simulink model "SWC_FDC_type"  (R2021b)
settings: Solver=FixedStepDiscrete  StartTime=0.0  StopTime=10.0  FixedStep=0.005  RelTol=1e-3
values from neighbouring files (symbols this model uses):
  FALSE = boolean( 0 )    [vcu_local_hdr.m]    (also in vcu_local_hdrTA2.m)
  TRUE = boolean( 1 )    [vcu_local_hdr.m]    (also in vcu_local_hdrTA2.m)
libraries: app x1
settings Model: DataDictionary=APPTypes.sldd  Creator=FVT22063  LastModifiedBy=zack
settings DataIOCC: SaveFormat=StructureWithTime
settings OptimizationCC: DefaultParameterBehavior=Inlined  EnhancedBackFolding=on  PassReuseOutputArgsAs=Individual arguments  ZeroExternalMemoryAtStartup=off  ZeroInternalMemoryAtStartup=off  OptimizeBlockOrder=speed  DifferentSizesBufferReuse=on  OptimizationCustomize=off  EfficientTunableParamExpr=on
settings DebuggingCC: ParameterTunabilityLossMsg=error
settings HardwareCC: ProdBitPerPointer=32  ProdBitPerSizeT=32  ProdBitPerPtrDiffT=32  ProdLargestAtomicInteger=Long  ProdLargestAtomicFloat=Double  ProdWordSize=32  ProdLongLongMode=on  ProdHWDeviceType=ARM Compatible->ARM Cortex-M
settings ModelReferenceCC: ModelReferenceNumInstancesAllowed=Single
settings SFSimCC: MATLABDynamicMemAlloc=off
settings RTWCC: Description=AUTOSAR  SystemTargetFile=autosar.tlc  GenCodeOnly=on  TemplateMakefile=ert_default_tmf  PortableWordSizes=on
settings CodeAppCC: ForceParamTrailComments=on  IgnoreCustomStorageClasses=off  OperatorAnnotations=on  SimulinkDataObjDesc=on  SFDataObjDesc=on  InsertBlockDesc=on
settings STFCustomTargetCC: TargetLangStandard=C99 (ISO)  MultiwordLength=256  ParMdlRefBuildCompliant=on  CompOptLevelCompliant=on  IncludeMdlTerminateFcn=off  CombineOutputUpdateFcns=on  SuppressErrorStatus=on  ERTCustomFileBanners=on  SupportNonFinite=off  SupportComplex=off  SupportContinuousTime=off  SupportNonInlinedSFcns=off  RemoveResetFunc=on  MATLABClassNameForMDSCustomization=Simulink.SoftwareTarget.ERTCustomization  AutosarCompliant=on  GRTInterface=off  UseToolchainInfoCompliant=on  LookupTableObjectStructAxisOrder=2,1,3,4,...  LUTObjectStructOrderEvenSpacing=Size,Table,Breakpoints  SystemTargetFile=autosar.tlc
settings ERTTargetCC: TargetLangStandard=C99 (ISO)  ConcurrentExecutionCompliant=off  IncludeMdlTerminateFcn=off  SuppressErrorStatus=on  SupportNonFinite=off  SupportComplex=off  ModelStepFunctionPrototypeControlCompliant=off  CPPClassGenCompliant=off  AutosarCompliant=on  LookupTableObjectStructAxisOrder=2,1,3,4,...  LUTObjectStructOrderEvenSpacing=Size,Table,Breakpoints  GenerateASAP2=on  InlinedParameterPlacement=NonHierarchical  ERTCustomFileTemplate=example_file_process.tlc  ConvertIfToSwitch=off  SuppressUnreachableDefaultCases=off  BooleanTrueId=true_MatlabRTW  BooleanFalseId=false_MatlabRTW

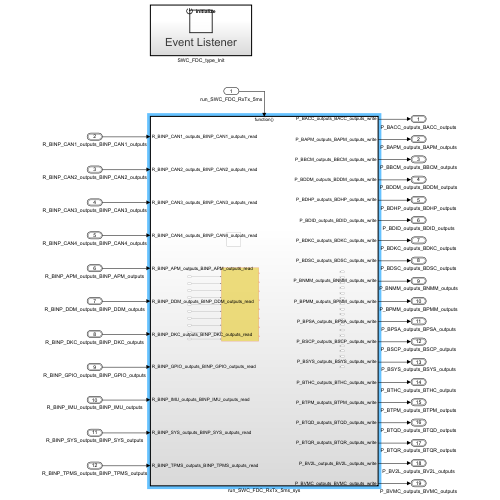
[thumbnail: Simulink's stored preview of the top-level diagram]
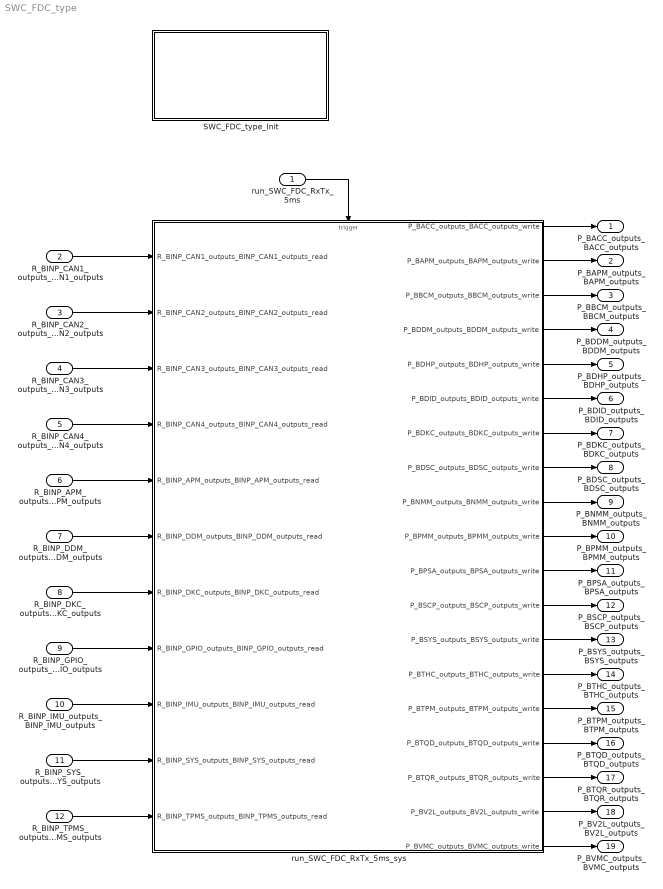
== system SWC_FDC_type ==
  run_SWC_FDC_RxTx_5ms : Inport  SampleTime=0.005  OutputFunctionCall=on
  R_BINP_CAN1_outputs_BINP_CAN1_outputs : Inport  Port=2  OutDataTypeStr=Bus: BINP_CAN1_outputs  PortDimensions=1  BusOutputAsStruct=on
  R_BINP_CAN2_outputs_BINP_CAN2_outputs : Inport  Port=3  OutDataTypeStr=Bus: BINP_CAN2_outputs  PortDimensions=1  BusOutputAsStruct=on
  R_BINP_CAN3_outputs_BINP_CAN3_outputs : Inport  Port=4  OutDataTypeStr=Bus: BINP_CAN3_outputs  PortDimensions=1  BusOutputAsStruct=on
  R_BINP_CAN4_outputs_BINP_CAN4_outputs : Inport  Port=5  OutDataTypeStr=Bus: BINP_CAN4_outputs  PortDimensions=1  BusOutputAsStruct=on
  R_BINP_APM_outputs_BINP_APM_outputs : Inport  Port=6  OutDataTypeStr=Bus: BINP_APM_outputs  PortDimensions=1  BusOutputAsStruct=on
  R_BINP_DDM_outputs_BINP_DDM_outputs : Inport  Port=7  OutDataTypeStr=Bus: BINP_DDM_outputs  PortDimensions=1  BusOutputAsStruct=on
  R_BINP_DKC_outputs_BINP_DKC_outputs : Inport  Port=8  OutDataTypeStr=Bus: BINP_DKC_outputs  PortDimensions=1  BusOutputAsStruct=on
  R_BINP_GPIO_outputs_BINP_GPIO_outputs : Inport  Port=9  OutDataTypeStr=Bus: BINP_GPIO_outputs  PortDimensions=1  BusOutputAsStruct=on
  R_BINP_IMU_outputs_BINP_IMU_outputs : Inport  Port=10  OutDataTypeStr=Bus: BINP_IMU_outputs  PortDimensions=1  BusOutputAsStruct=on
  R_BINP_SYS_outputs_BINP_SYS_outputs : Inport  Port=11  OutDataTypeStr=Bus: BINP_SYS_outputs  PortDimensions=1  BusOutputAsStruct=on
  R_BINP_TPMS_outputs_BINP_TPMS_outputs : Inport  Port=12  OutDataTypeStr=Bus: BINP_TPMS_outputs  PortDimensions=1  BusOutputAsStruct=on
  SWC_FDC_type_Init : Subsystem
  run_SWC_FDC_RxTx_5ms_sys : Subsystem
  P_BACC_outputs_BACC_outputs : Outport  OutDataTypeStr=Bus: BACC_outputs  PortDimensions=1  BusOutputAsStruct=on
  P_BAPM_outputs_BAPM_outputs : Outport  Port=2  OutDataTypeStr=Bus: BAPM_outputs  PortDimensions=1  BusOutputAsStruct=on
  P_BBCM_outputs_BBCM_outputs : Outport  Port=3  OutDataTypeStr=Bus: BBCM_outputs  PortDimensions=1  BusOutputAsStruct=on
  P_BDDM_outputs_BDDM_outputs : Outport  Port=4  OutDataTypeStr=Bus: BDDM_outputs  PortDimensions=1  BusOutputAsStruct=on
  P_BDHP_outputs_BDHP_outputs : Outport  Port=5  OutDataTypeStr=Bus: BDHP_outputs  PortDimensions=1  BusOutputAsStruct=on
  P_BDID_outputs_BDID_outputs : Outport  Port=6  OutDataTypeStr=Bus: BDID_outputs  PortDimensions=1  BusOutputAsStruct=on
  P_BDKC_outputs_BDKC_outputs : Outport  Port=7  OutDataTypeStr=Bus: BDKC_outputs  PortDimensions=1  BusOutputAsStruct=on
  P_BDSC_outputs_BDSC_outputs : Outport  Port=8  OutDataTypeStr=Bus: BDSC_outputs  PortDimensions=1  BusOutputAsStruct=on
  P_BNMM_outputs_BNMM_outputs : Outport  Port=9  OutDataTypeStr=Bus: BNMM_outputs  PortDimensions=1  BusOutputAsStruct=on
  P_BPMM_outputs_BPMM_outputs : Outport  Port=10  OutDataTypeStr=Bus: BPMM_outputs  PortDimensions=1  BusOutputAsStruct=on
  P_BPSA_outputs_BPSA_outputs : Outport  Port=11  OutDataTypeStr=Bus: BPSA_outputs  PortDimensions=1  BusOutputAsStruct=on
  P_BSCP_outputs_BSCP_outputs : Outport  Port=12  OutDataTypeStr=Bus: BSCP_outputs  PortDimensions=1  BusOutputAsStruct=on
  P_BSYS_outputs_BSYS_outputs : Outport  Port=13  OutDataTypeStr=Bus: BSYS_outputs  PortDimensions=1  BusOutputAsStruct=on
  P_BTHC_outputs_BTHC_outputs : Outport  Port=14  OutDataTypeStr=Bus: BTHC_outputs  PortDimensions=1  BusOutputAsStruct=on
  P_BTPM_outputs_BTPM_outputs : Outport  Port=15  OutDataTypeStr=Bus: BTPM_outputs  PortDimensions=1  BusOutputAsStruct=on
  P_BTQD_outputs_BTQD_outputs : Outport  Port=16  OutDataTypeStr=Bus: BTQD_outputs  PortDimensions=1  BusOutputAsStruct=on
  P_BTQR_outputs_BTQR_outputs : Outport  Port=17  OutDataTypeStr=Bus: BTQR_outputs  PortDimensions=1  BusOutputAsStruct=on
  P_BV2L_outputs_BV2L_outputs : Outport  Port=18  OutDataTypeStr=Bus: BV2L_outputs  PortDimensions=1  BusOutputAsStruct=on
  P_BVMC_outputs_BVMC_outputs : Outport  Port=19  OutDataTypeStr=Bus: BVMC_outputs  PortDimensions=1  BusOutputAsStruct=on
  wires:
  R_BINP_CAN1_outputs_BINP_CAN1_outputs/1 -> run_SWC_FDC_RxTx_5ms_sys/1(R_BINP_CAN1_outputs_BINP_CAN1_outputs_read)
  R_BINP_CAN2_outputs_BINP_CAN2_outputs/1 -> run_SWC_FDC_RxTx_5ms_sys/2(R_BINP_CAN2_outputs_BINP_CAN2_outputs_read)
  R_BINP_CAN3_outputs_BINP_CAN3_outputs/1 -> run_SWC_FDC_RxTx_5ms_sys/3(R_BINP_CAN3_outputs_BINP_CAN3_outputs_read)
  R_BINP_CAN4_outputs_BINP_CAN4_outputs/1 -> run_SWC_FDC_RxTx_5ms_sys/4(R_BINP_CAN4_outputs_BINP_CAN4_outputs_read)
  R_BINP_APM_outputs_BINP_APM_outputs/1 -> run_SWC_FDC_RxTx_5ms_sys/5(R_BINP_APM_outputs_BINP_APM_outputs_read)
  R_BINP_DDM_outputs_BINP_DDM_outputs/1 -> run_SWC_FDC_RxTx_5ms_sys/6(R_BINP_DDM_outputs_BINP_DDM_outputs_read)
  R_BINP_DKC_outputs_BINP_DKC_outputs/1 -> run_SWC_FDC_RxTx_5ms_sys/7(R_BINP_DKC_outputs_BINP_DKC_outputs_read)
  R_BINP_GPIO_outputs_BINP_GPIO_outputs/1 -> run_SWC_FDC_RxTx_5ms_sys/8(R_BINP_GPIO_outputs_BINP_GPIO_outputs_read)
  R_BINP_IMU_outputs_BINP_IMU_outputs/1 -> run_SWC_FDC_RxTx_5ms_sys/9(R_BINP_IMU_outputs_BINP_IMU_outputs_read)
  R_BINP_SYS_outputs_BINP_SYS_outputs/1 -> run_SWC_FDC_RxTx_5ms_sys/10(R_BINP_SYS_outputs_BINP_SYS_outputs_read)
  R_BINP_TPMS_outputs_BINP_TPMS_outputs/1 -> run_SWC_FDC_RxTx_5ms_sys/11(R_BINP_TPMS_outputs_BINP_TPMS_outputs_read)
  run_SWC_FDC_RxTx_5ms_sys/1(P_BACC_outputs_BACC_outputs_write) -> P_BACC_outputs_BACC_outputs/1
  run_SWC_FDC_RxTx_5ms_sys/2(P_BAPM_outputs_BAPM_outputs_write) -> P_BAPM_outputs_BAPM_outputs/1
  run_SWC_FDC_RxTx_5ms_sys/3(P_BBCM_outputs_BBCM_outputs_write) -> P_BBCM_outputs_BBCM_outputs/1
  run_SWC_FDC_RxTx_5ms_sys/4(P_BDDM_outputs_BDDM_outputs_write) -> P_BDDM_outputs_BDDM_outputs/1
  run_SWC_FDC_RxTx_5ms_sys/5(P_BDHP_outputs_BDHP_outputs_write) -> P_BDHP_outputs_BDHP_outputs/1
  run_SWC_FDC_RxTx_5ms_sys/6(P_BDID_outputs_BDID_outputs_write) -> P_BDID_outputs_BDID_outputs/1
  run_SWC_FDC_RxTx_5ms_sys/7(P_BDKC_outputs_BDKC_outputs_write) -> P_BDKC_outputs_BDKC_outputs/1
  run_SWC_FDC_RxTx_5ms_sys/8(P_BDSC_outputs_BDSC_outputs_write) -> P_BDSC_outputs_BDSC_outputs/1
  run_SWC_FDC_RxTx_5ms_sys/9(P_BNMM_outputs_BNMM_outputs_write) -> P_BNMM_outputs_BNMM_outputs/1
  run_SWC_FDC_RxTx_5ms_sys/10(P_BPMM_outputs_BPMM_outputs_write) -> P_BPMM_outputs_BPMM_outputs/1
  run_SWC_FDC_RxTx_5ms_sys/11(P_BPSA_outputs_BPSA_outputs_write) -> P_BPSA_outputs_BPSA_outputs/1
  run_SWC_FDC_RxTx_5ms_sys/12(P_BSCP_outputs_BSCP_outputs_write) -> P_BSCP_outputs_BSCP_outputs/1
  run_SWC_FDC_RxTx_5ms_sys/13(P_BSYS_outputs_BSYS_outputs_write) -> P_BSYS_outputs_BSYS_outputs/1
  run_SWC_FDC_RxTx_5ms_sys/14(P_BTHC_outputs_BTHC_outputs_write) -> P_BTHC_outputs_BTHC_outputs/1
  run_SWC_FDC_RxTx_5ms_sys/15(P_BTPM_outputs_BTPM_outputs_write) -> P_BTPM_outputs_BTPM_outputs/1
  run_SWC_FDC_RxTx_5ms_sys/16(P_BTQD_outputs_BTQD_outputs_write) -> P_BTQD_outputs_BTQD_outputs/1
  run_SWC_FDC_RxTx_5ms_sys/17(P_BTQR_outputs_BTQR_outputs_write) -> P_BTQR_outputs_BTQR_outputs/1
  run_SWC_FDC_RxTx_5ms_sys/18(P_BV2L_outputs_BV2L_outputs_write) -> P_BV2L_outputs_BV2L_outputs/1
  run_SWC_FDC_RxTx_5ms_sys/19(P_BVMC_outputs_BVMC_outputs_write) -> P_BVMC_outputs_BVMC_outputs/1
  run_SWC_FDC_RxTx_5ms/1 -> run_SWC_FDC_RxTx_5ms_sys/Trigger

== system SWC_FDC_type/SWC_FDC_type_Init ==
  Event Listener : EventListener  EventName=reset

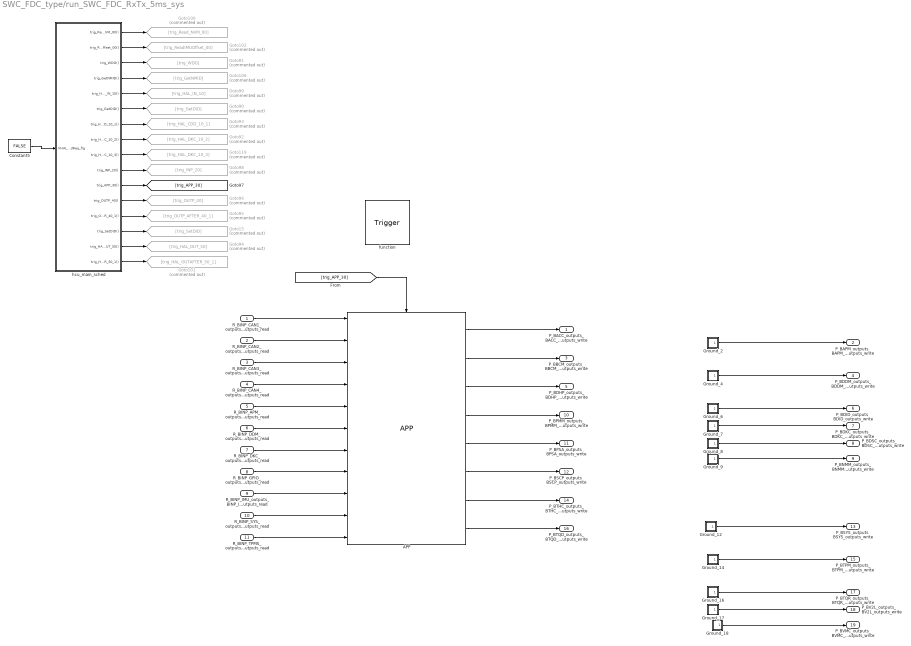
== system SWC_FDC_type/run_SWC_FDC_RxTx_5ms_sys ==
  R_BINP_CAN1_outputs_BINP_CAN1_outputs_read : Inport
  R_BINP_CAN2_outputs_BINP_CAN2_outputs_read : Inport  Port=2
  R_BINP_CAN3_outputs_BINP_CAN3_outputs_read : Inport  Port=3
  R_BINP_CAN4_outputs_BINP_CAN4_outputs_read : Inport  Port=4
  R_BINP_APM_outputs_BINP_APM_outputs_read : Inport  Port=5
  R_BINP_DDM_outputs_BINP_DDM_outputs_read : Inport  Port=6
  R_BINP_DKC_outputs_BINP_DKC_outputs_read : Inport  Port=7
  R_BINP_GPIO_outputs_BINP_GPIO_outputs_read : Inport  Port=8
  R_BINP_IMU_outputs_BINP_IMU_outputs_read : Inport  Port=9
  R_BINP_SYS_outputs_BINP_SYS_outputs_read : Inport  Port=10
  R_BINP_TPMS_outputs_BINP_TPMS_outputs_read : Inport  Port=11
  function : TriggerPort  TriggerType=function-call  VariantControl=(inherit)  SampleTimeType=periodic  SampleTime=-1
  APP : app/APP  SystemSampleTime=-1  VariantActivationTime=update diagram  Latency=0  AutoFrameSizeCalculation=off
  Constant5 : Constant  Value=FALSE
  Goto100 : Goto  Commented=on  GotoTag=trig_Read_NVM_00
  Goto101 : Goto  Commented=on  GotoTag=trig_HAL_OUTAFTER_50_1
  Goto102 : Goto  Commented=on  GotoTag=trig_ReadIMUOffset_00
  Goto106 : Goto  Commented=on  GotoTag=trig_GetNMID
  Goto119 : Goto  Commented=on  GotoTag=trig_HAL_DKC_10_3
  Goto15 : Goto  Commented=on  GotoTag=trig_SetDID
  Goto90 : Goto  Commented=on  GotoTag=trig_GetDID
  Goto91 : Goto  Commented=on  GotoTag=trig_WDG
  Goto92 : Goto  Commented=on  GotoTag=trig_HAL_DKC_10_2
  Goto93 : Goto  Commented=on  GotoTag=trig_HAL_CDD_10_1
  Goto94 : Goto  Commented=on  GotoTag=trig_HAL_OUT_50
  Goto95 : Goto  Commented=on  GotoTag=trig_OUTP_AFTER_40_1
  Goto96 : Goto  Commented=on  GotoTag=trig_OUTP_40
  Goto98 : Goto  Commented=on  GotoTag=trig_INP_20
  Goto99 : Goto  Commented=on  GotoTag=trig_HAL_IN_10
  Ground_12 : Subsystem
  Ground_14 : Subsystem
  Ground_16 : Subsystem
  Ground_17 : Subsystem
  Ground_18 : Subsystem
  Ground_2 : Subsystem
  Ground_4 : Subsystem
  Ground_6 : Subsystem
  Ground_7 : Subsystem
  Ground_8 : Subsystem
  Ground_9 : Subsystem
  hcu_main_sched : Stateflow chart  TreatAsAtomicUnit=on
  P_BACC_outputs_BACC_outputs_write : Outport
  P_BAPM_outputs_BAPM_outputs_write : Outport  Port=2
  P_BBCM_outputs_BBCM_outputs_write : Outport  Port=3
  P_BDDM_outputs_BDDM_outputs_write : Outport  Port=4
  P_BDHP_outputs_BDHP_outputs_write : Outport  Port=5
  P_BDID_outputs_BDID_outputs_write : Outport  Port=6
  P_BDKC_outputs_BDKC_outputs_write : Outport  Port=7
  P_BDSC_outputs_BDSC_outputs_write : Outport  Port=8
  P_BNMM_outputs_BNMM_outputs_write : Outport  Port=9
  P_BPMM_outputs_BPMM_outputs_write : Outport  Port=10
  P_BPSA_outputs_BPSA_outputs_write : Outport  Port=11
  P_BSCP_outputs_BSCP_outputs_write : Outport  Port=12
  P_BSYS_outputs_BSYS_outputs_write : Outport  Port=13
  P_BTHC_outputs_BTHC_outputs_write : Outport  Port=14
  P_BTPM_outputs_BTPM_outputs_write : Outport  Port=15
  P_BTQD_outputs_BTQD_outputs_write : Outport  Port=16
  P_BTQR_outputs_BTQR_outputs_write : Outport  Port=17
  P_BV2L_outputs_BV2L_outputs_write : Outport  Port=18
  P_BVMC_outputs_BVMC_outputs_write : Outport  Port=19
  wires:
  R_BINP_CAN2_outputs_BINP_CAN2_outputs_read/1 -> APP/2
  R_BINP_CAN3_outputs_BINP_CAN3_outputs_read/1 -> APP/3
  R_BINP_CAN1_outputs_BINP_CAN1_outputs_read/1 -> APP/1
  R_BINP_CAN4_outputs_BINP_CAN4_outputs_read/1 -> APP/4
  R_BINP_APM_outputs_BINP_APM_outputs_read/1 -> APP/5
  R_BINP_DDM_outputs_BINP_DDM_outputs_read/1 -> APP/6
  R_BINP_DKC_outputs_BINP_DKC_outputs_read/1 -> APP/7
  R_BINP_GPIO_outputs_BINP_GPIO_outputs_read/1 -> APP/8
  R_BINP_IMU_outputs_BINP_IMU_outputs_read/1 -> APP/9
  R_BINP_SYS_outputs_BINP_SYS_outputs_read/1 -> APP/10
  R_BINP_TPMS_outputs_BINP_TPMS_outputs_read/1 -> APP/11
  hcu_main_sched/4(trig_GetNMID()) -> Goto106/1
  hcu_main_sched/12(trig_OUTP_40()) -> Goto96/1
  hcu_main_sched/13(trig_OUTP_AFTER_40_1()) -> Goto95/1
  hcu_main_sched/3(trig_WDG()) -> Goto91/1
  hcu_main_sched/9(trig_HAL_DKC_10_3()) -> Goto119/1
  hcu_main_sched/2(trig_ReadIMUOffset_00()) -> Goto102/1
  hcu_main_sched/16(trig_HAL_OUTAFTER_50_1()) -> Goto101/1
  hcu_main_sched/14(trig_SetDID()) -> Goto15/1
  hcu_main_sched/15(trig_HAL_OUT_50()) -> Goto94/1
  hcu_main_sched/7(trig_HAL_CDD_10_1()) -> Goto93/1
  Constant5/1 -> hcu_main_sched/1(VHAL_FusionSchedReq_flg)
  hcu_main_sched/11(trig_APP_30()) -> [trig_APP_30]
  hcu_main_sched/6(trig_GetDID()) -> Goto90/1
  hcu_main_sched/1(trig_Read_NVM_00()) -> Goto100/1
  hcu_main_sched/5(trig_HAL_IN_10()) -> Goto99/1
  hcu_main_sched/8(trig_HAL_DKC_10_2()) -> Goto92/1
  hcu_main_sched/10(trig_INP_20()) -> Goto98/1
  APP/1 -> P_BACC_outputs_BACC_outputs_write/1
  APP/2 -> P_BBCM_outputs_BBCM_outputs_write/1
  APP/3 -> P_BDHP_outputs_BDHP_outputs_write/1
  APP/4 -> P_BPMM_outputs_BPMM_outputs_write/1
  APP/5 -> P_BPSA_outputs_BPSA_outputs_write/1
  APP/6 -> P_BSCP_outputs_BSCP_outputs_write/1
  APP/7 -> P_BTHC_outputs_BTHC_outputs_write/1
  APP/8 -> P_BTQD_outputs_BTQD_outputs_write/1
  Ground_2/1(P_BAPM_outputs_BAPM_outputs_write) -> P_BAPM_outputs_BAPM_outputs_write/1
  Ground_8/1(P_BDSC_outputs_BDSC_outputs_write) -> P_BDSC_outputs_BDSC_outputs_write/1
  Ground_17/1(Out1) -> P_BV2L_outputs_BV2L_outputs_write/1
  Ground_7/1(P_BDKC_outputs_BDKC_outputs_write) -> P_BDKC_outputs_BDKC_outputs_write/1
  Ground_18/1(P_BVMC_outputs_BVMC_outputs_write) -> P_BVMC_outputs_BVMC_outputs_write/1
  Ground_6/1(P_BDID_outputs_BDID_outputs_write) -> P_BDID_outputs_BDID_outputs_write/1
  Ground_4/1(P_BDDM_outputs_BDDM_outputs_write) -> P_BDDM_outputs_BDDM_outputs_write/1
  Ground_14/1(Out1) -> P_BTPM_outputs_BTPM_outputs_write/1
  Ground_16/1(Out1) -> P_BTQR_outputs_BTQR_outputs_write/1
  Ground_12/1(Out1) -> P_BSYS_outputs_BSYS_outputs_write/1
  Ground_9/1(P_BNMM_outputs_BNMM_outputs_write) -> P_BNMM_outputs_BNMM_outputs_write/1
  [trig_APP_30] -> APP/Trigger

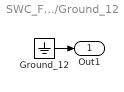
== system SWC_FDC_type/run_SWC_FDC_RxTx_5ms_sys/Ground_12 ==
  Ground_12 : Ground
  Out1 : Outport  OutDataTypeStr=Bus: BSYS_outputs  PortDimensions=1
  wires:
  Ground_12/1 -> Out1/1

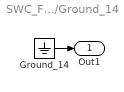
== system SWC_FDC_type/run_SWC_FDC_RxTx_5ms_sys/Ground_14 ==
  Ground_14 : Ground
  Out1 : Outport  OutDataTypeStr=Bus: BTPM_outputs  PortDimensions=1
  wires:
  Ground_14/1 -> Out1/1

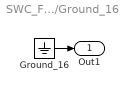
== system SWC_FDC_type/run_SWC_FDC_RxTx_5ms_sys/Ground_16 ==
  Ground_16 : Ground
  Out1 : Outport  OutDataTypeStr=Bus: BTQR_outputs  PortDimensions=1
  wires:
  Ground_16/1 -> Out1/1

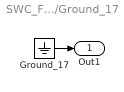
== system SWC_FDC_type/run_SWC_FDC_RxTx_5ms_sys/Ground_17 ==
  Ground_17 : Ground
  Out1 : Outport  OutDataTypeStr=Bus: BV2L_outputs  PortDimensions=1
  wires:
  Ground_17/1 -> Out1/1

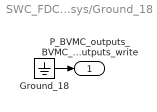
== system SWC_FDC_type/run_SWC_FDC_RxTx_5ms_sys/Ground_18 ==
  Ground_18 : Ground
  P_BVMC_outputs_BVMC_outputs_write : Outport  OutDataTypeStr=Bus: BVMC_outputs  PortDimensions=1
  wires:
  Ground_18/1 -> P_BVMC_outputs_BVMC_outputs_write/1

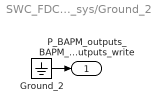
== system SWC_FDC_type/run_SWC_FDC_RxTx_5ms_sys/Ground_2 ==
  Ground_2 : Ground
  P_BAPM_outputs_BAPM_outputs_write : Outport  OutDataTypeStr=Bus: BAPM_outputs  PortDimensions=1
  wires:
  Ground_2/1 -> P_BAPM_outputs_BAPM_outputs_write/1

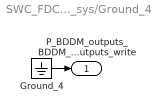
== system SWC_FDC_type/run_SWC_FDC_RxTx_5ms_sys/Ground_4 ==
  Ground_4 : Ground
  P_BDDM_outputs_BDDM_outputs_write : Outport  OutDataTypeStr=Bus: BDDM_outputs  PortDimensions=1
  wires:
  Ground_4/1 -> P_BDDM_outputs_BDDM_outputs_write/1

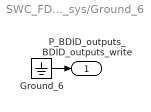
== system SWC_FDC_type/run_SWC_FDC_RxTx_5ms_sys/Ground_6 ==
  Ground_6 : Ground
  P_BDID_outputs_BDID_outputs_write : Outport  OutDataTypeStr=Bus: BDID_outputs  PortDimensions=1
  wires:
  Ground_6/1 -> P_BDID_outputs_BDID_outputs_write/1

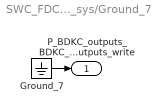
== system SWC_FDC_type/run_SWC_FDC_RxTx_5ms_sys/Ground_7 ==
  Ground_7 : Ground
  P_BDKC_outputs_BDKC_outputs_write : Outport  OutDataTypeStr=Bus: BDKC_outputs  PortDimensions=1
  wires:
  Ground_7/1 -> P_BDKC_outputs_BDKC_outputs_write/1

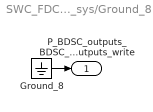
== system SWC_FDC_type/run_SWC_FDC_RxTx_5ms_sys/Ground_8 ==
  Ground_8 : Ground
  P_BDSC_outputs_BDSC_outputs_write : Outport  OutDataTypeStr=Bus: BDSC_outputs  PortDimensions=1
  wires:
  Ground_8/1 -> P_BDSC_outputs_BDSC_outputs_write/1

== system SWC_FDC_type/run_SWC_FDC_RxTx_5ms_sys/Ground_9 ==
  Ground_9 : Ground
  P_BNMM_outputs_BNMM_outputs_write : Outport  OutDataTypeStr=Bus: BNMM_outputs  PortDimensions=1
  wires:
  Ground_9/1 -> P_BNMM_outputs_BNMM_outputs_write/1

== stateflow chart SWC_FDC_type/run_SWC_FDC_RxTx_5ms_sys/hcu_main_sched ==
  state Main_Scheduler
    (default) -> (junction 31) : {
        |   Sys_Init_done = FALSE;
        |   trig_Read_NVM_00;
        |   trig_ReadIMUOffset_00;
        | }
    Main_Scheduler -> (junction 31) : {Sys_Init_done = TRUE;}
    (junction 31) -> (junction 34) [order 1] : [
        |    Sys_Init_done &&...
        |    !VHAL_FusionSchedReq_flg
        | ]
    (junction 31) -> (junction 38) [order 2]
    (junction 34) -> (junction 36) : {
        |     trig_WDG;
        |     trig_GetNMID;
        |     trig_HAL_IN_10;
        |     trig_GetDID;
        |     trig_HAL_CDD_10_1;
        |     trig_HAL_DKC_10_2;
        |     trig_HAL_DKC_10_3;
        |     trig_INP_20;
        |     trig_APP_30;
        |     trig_OUTP_40;
        |     trig_OUTP_AFTER_40_1;
        |     trig_SetDID;
        |     trig_HAL_OUT_50;
        |     trig_HAL_OUTAFTER_50_1;
        |    }
    (junction 36) -> (junction 38)
  (default) -> Main_Scheduler
  data: VHAL_FusionSchedReq_flg input; Sys_Init_done local double; FALSE parameter; TRUE parameter
  events: trig_Read_NVM_00 output FUNCTION_CALL_EVENT; trig_ReadIMUOffset_00 output FUNCTION_CALL_EVENT; trig_WDG output FUNCTION_CALL_EVENT; trig_GetNMID output FUNCTION_CALL_EVENT; trig_HAL_IN_10 output FUNCTION_CALL_EVENT; trig_GetDID output FUNCTION_CALL_EVENT; trig_HAL_CDD_10_1 output FUNCTION_CALL_EVENT; trig_HAL_DKC_10_2 output FUNCTION_CALL_EVENT; trig_HAL_DKC_10_3 output FUNCTION_CALL_EVENT; trig_INP_20 output FUNCTION_CALL_EVENT; trig_APP_30 output FUNCTION_CALL_EVENT; trig_OUTP_40 output FUNCTION_CALL_EVENT; trig_OUTP_AFTER_40_1 output FUNCTION_CALL_EVENT; trig_SetDID output FUNCTION_CALL_EVENT; trig_HAL_OUT_50 output FUNCTION_CALL_EVENT; trig_HAL_OUTAFTER_50_1 output FUNCTION_CALL_EVENT
